simulink model "lane_select"  (R2016b)
settings: Solver=VariableStepAuto  StartTime=0.0  StopTime=10.0  RelTol=1e-3
libraries: robotlib x4
settings Model: Creator=shota  LastModifiedBy=shota

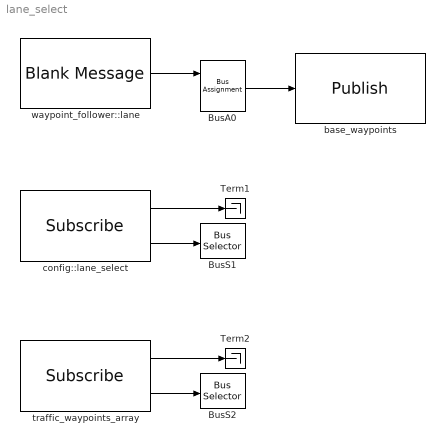
== system lane_select ==
  BusA0 : BusAssignment  AssignedSignals=signal1
  BusS1 : BusSelector  OutputSignals=signal1,signal2
  BusS2 : BusSelector  OutputSignals=signal1,signal2
  Term1 : Terminator
  Term2 : Terminator
  base_waypoints : robotlib/Publish  SourceLibraryInfo=This block requires Robotics System Toolbox  topicSource=Specify your own  topic=/base_waypoints  messageType=waypoint_follower/lane  messageQueueLength=1
  config::lane_select : robotlib/Subscribe  SourceLibraryInfo=This block requires Robotics System Toolbox  topicSource=Specify your own  topic=/config/lane_select  messageType=runtime_manager/ConfigLaneSelect  sampleTime=-1  messageQueueLength=1
  traffic_waypoints_array : robotlib/Subscribe  SourceLibraryInfo=This block requires Robotics System Toolbox  topicSource=Specify your own  topic=/traffic_waypoints_array  messageType=waypoint_follower/LaneArray  sampleTime=-1  messageQueueLength=1
  waypoint_follower::lane : robotlib/Blank Message  SourceLibraryInfo=This block requires Robotics System Toolbox  messageType=waypoint_follower/lane  SampleTime=inf
  wires:
  waypoint_follower::lane/1 -> BusA0/1
  BusA0/1 -> base_waypoints/1
  config::lane_select/1 -> Term1/1
  config::lane_select/2 -> BusS1/1
  traffic_waypoints_array/1 -> Term2/1
  traffic_waypoints_array/2 -> BusS2/1
